simulink model "NonLinearODESim"  (R2025a)
settings: Solver=ode4  StartTime=0.0  StopTime=inf  FixedStep=0.01  RelTol=1e-3
settings Model: Creator=bulve  LastModifiedBy=BjørnErikUlveraker

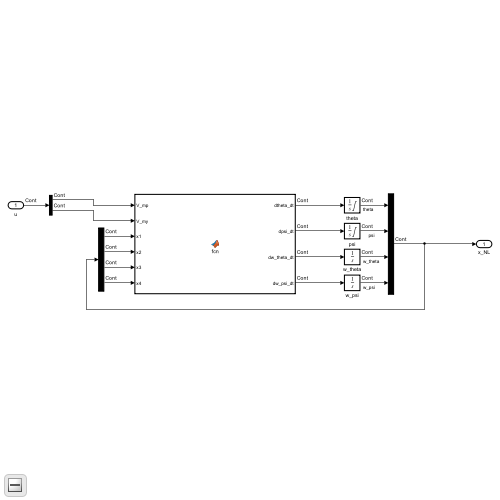
[thumbnail: Simulink's stored preview of the top-level diagram]
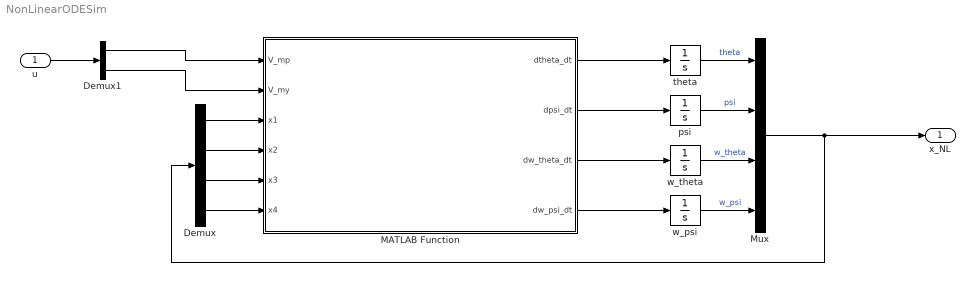
== system NonLinearODESim ==
  u : Inport
  Demux : Demux
  Demux1 : Demux  Outputs=2
  MATLAB Function : MATLAB Function  TreatAsAtomicUnit=on
  Mux : Mux
  psi : Integrator  InitialCondition=pi/2  LimitOutput=on  UpperSaturationLimit=pi  LowerSaturationLimit=0
  theta : Integrator  InitialCondition=-10*pi/180  LimitOutput=on  UpperSaturationLimit=45*pi/180  LowerSaturationLimit=-45*pi/180
  w_psi : Integrator
  w_theta : Integrator
  x_NL : Outport
  wires:
  MATLAB Function/1(dtheta_dt) -> theta/1
  MATLAB Function/2(dpsi_dt) -> psi/1
  MATLAB Function/3(dw_theta_dt) -> w_theta/1
  MATLAB Function/4(dw_psi_dt) -> w_psi/1
  theta/1 -> Mux/1  "theta"
  psi/1 -> Mux/2  "psi"
  w_theta/1 -> Mux/3  "w_theta"
  w_psi/1 -> Mux/4  "w_psi"
  Demux/4 -> MATLAB Function/6(x4)
  Demux/3 -> MATLAB Function/5(x3)
  Demux/2 -> MATLAB Function/4(x2)
  Demux/1 -> MATLAB Function/3(x1)
  u/1 -> Demux1/1
  Demux1/1 -> MATLAB Function/1(V_mp)
  Demux1/2 -> MATLAB Function/2(V_my)
  Mux/1 -> x_NL/1, Demux/1

== matlab function NonLinearODESim/MATLAB Function ==
  data: V_mp input; V_my input; x1 input; dtheta_dt output; x2 input; x3 input; x4 input; dpsi_dt output; dw_theta_dt output; dw_psi_dt output
function [dtheta_dt,dpsi_dt,dw_theta_dt,dw_psi_dt] = fcn(V_mp, V_my,x1,x2,x3,x4)

%States
theta = x1;
psi= x2; 
w_theta=x3;
w_psi=x4;

%Parameters
l_cm = 0.015; %[m]
m_heli = 0.479; %[kg]
J_eq_p = 0.0172; %[kg*m^2]
J_eq_y = 0.0210; %[kg*m^2]
g = 9.81; %[m*s^2]

K_pp = 0.0556; %[Nm/V]
K_yy = 0.21084; %[Nm/V]
K_py = 0.005; %[Nm/V]
K_yp = 0.15; %[Nm/V]
B_p = 0.01; %[N/V]
B_y = 0.08; %[N/V]


% Common denominatorsa
Dp = J_eq_p + m_heli*l_cm.^2;
Dy = J_eq_y + m_heli*l_cm.^2.*cos(theta).^2;

%Differential equations 
dtheta_dt = w_theta;

dpsi_dt = w_psi;

dw_theta_dt = (K_pp*V_mp)/Dp-(K_py*V_my)/Dp-(B_p*w_theta+m_heli*w_psi.^2*sin(theta)*l_cm^2*cos(theta)+m_heli*g*cos(theta)*l_cm)/Dp;

dw_psi_dt = (K_yp*V_mp)/Dy-(K_yy*V_my)/Dy+(2*m_heli*w_psi*sin(theta)*l_cm.^2*cos(theta)*w_theta)/Dy-(B_y*w_psi)/Dy;
